simulink library "MotorLIB"  (R2019a)
settings: Solver=VariableStepAuto  StartTime=0.0  StopTime=10.0  RelTol=1e-3
libraries: fl_lib x5, nesl_utility x2, ee_lib x1
settings Model: Creator=plewi  LastModifiedBy=plewi

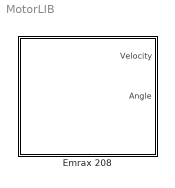
== system MotorLIB ==
  Emrax 208 : Subsystem  mask(Emrax 208){nPolePairs=10, pm_flux_linkage=0.05, Ld=125e-6, Lq=130e-6, L0=2e-4, Rs=0.35, J=256e3}
      mask prompts: nPolePairs "Number of pole pairs"; pm_flux_linkage "Permanent magnet flux linkage"; Ld "Stator d-axis inductance, Ld"; Lq "Stator q-axis inductance, Lq"; L0 "Stator zero-sequence inductance, L0"; Rs "Stator resistance per phase, Rs"; J "Rotor inertia (g cm^2)"
      mask help: Permanent Magnet Synchronous Motor with resolver attachment.
      mask TypeOptions nPolePairs:
      | Permanent Magnet
      | Synchronous Motor/nPolePairs
      mask TypeOptions pm_flux_linkage:
      | Permanent Magnet
      | Synchronous Motor/pm_flux_linkage
      mask TypeOptions Ld:
      | Permanent Magnet
      | Synchronous Motor/Ld
      mask TypeOptions Lq:
      | Permanent Magnet
      | Synchronous Motor/Lq
      mask TypeOptions L0:
      | Permanent Magnet
      | Synchronous Motor/L0
      mask TypeOptions Rs:
      | Permanent Magnet
      | Synchronous Motor/Rs
      mask TypeOptions J:
      | Permanent Magnet
      | Synchronous Motor/J
      mask Display: image('C:\Users\plewi\Documents\University\6-Sixth Year\MUR\MUR-E_Simulation_2019\Images\emrax_208_ip65_01-1-1024x1024.jpg');

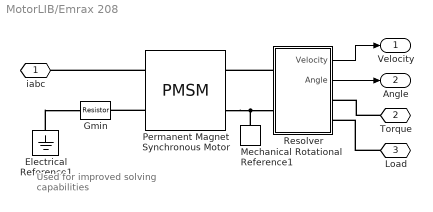
== system MotorLIB/Emrax 208 ==
  note: Used for improved
      | solving capabilities
  Electrical Reference1 : fl_lib/Electrical/Electrical Elements/Electrical Reference
  Gmin : fl_lib/Electrical/Electrical Elements/Resistor  R=1e9 Ohm  i_specify=off  i_priority=High  i=0 A  i_nominal_specify=off  i_nominal_unit=A  i_nominal_value=1  v_specify=off  v_priority=High  v=0 V  v_nominal_specify=off  v_nominal_unit=V  v_nominal_value=1
  Mechanical Rotational Reference1 : fl_lib/Mechanical/Rotational Elements/Mechanical Rotational Reference
  Permanent Magnet Synchronous Motor : ee_lib/Electromechanical/Permanent Magnet/PMSM  nPolePairs=nPolePairs  pmflux_param=1  pm_flux_linkage=pm_flux_linkage Wb  torque_constant=0.18 N*m/A  back_emf_constant=0.18 V/(rad/s)  stator_param=1  Ld=Ld H  Lq=Lq H  L0=L0 H  Ls=0.0002 H  Lm=0.00002 H  Ms=0.00002 H  Rs=Rs Ohm  zero_sequence=ee.enum.park.zerosequence.include  J=J g*cm^2  lam=0.01 N*m/(rad/s)  axes_param=ee.enum.rotorangle.qaxis  i_d_specify=off  i_d_priority=None  i_d=0 A  i_d_nominal_specify=off  i_d_nominal_unit=A  i_d_nominal_value=1  i_q_specify=off  i_q_priority=None  i_q=0 A  i_q_nominal_specify=off  i_q_nominal_unit=A  i_q_nominal_value=1  torque_specify=off  torque_priority=None  torque=0 N*m  torque_nominal_specify=off  torque_nominal_unit=N*m  torque_nominal_value=1  angular_velocity_specify=on  angular_velocity_priority=High  angular_velocity=0 rpm  angular_velocity_nominal_specify=off  angular_velocity_nominal_unit=rpm  angular_velocity_nominal_value=1  angular_position_specify=on  angular_position_priority=High  angular_position=0 rad  angular_position_nominal_specify=off  angular_position_nominal_unit=deg  angular_position_nominal_value=1  mask(PMSM){}
      settings: SourceProductName=Simscape Electrical
  Resolver : Subsystem
  iabc : PMIOPort  Side=Left
  Torque : PMIOPort  Port=2  Side=Right
  Load : PMIOPort  Port=3  Side=Left
  Velocity : Outport
  Angle : Outport  Port=2
  wires:
  Resolver/1(Velocity) -> Velocity/1
  Resolver/2(Angle) -> Angle/1
  connections:
  Electrical Reference1/LConn1 -- Gmin/LConn1
  Mechanical Rotational Reference1/LConn1 -- Permanent Magnet Synchronous Motor/RConn2 -- Resolver/LConn2
  Load/RConn1 -- Resolver/RConn2
  Permanent Magnet Synchronous Motor/LConn2 -- Gmin/RConn1
  Resolver/LConn1 -- Permanent Magnet Synchronous Motor/RConn1
  Permanent Magnet Synchronous Motor/LConn1 -- iabc/RConn1
  Torque/RConn1 -- Resolver/RConn1

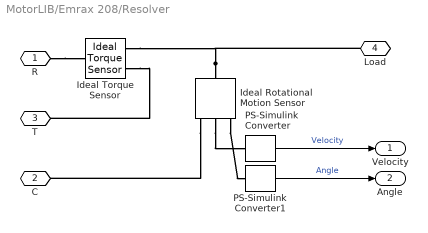
== system MotorLIB/Emrax 208/Resolver ==
  Ideal Rotational Motion Sensor : fl_lib/Mechanical/Mechanical Sensors/Ideal Rotational Motion Sensor  offset=0 deg
      settings: SourceProductName=Foundation Library
  Ideal Torque Sensor : fl_lib/Mechanical/Mechanical Sensors/Ideal Torque Sensor
      settings: SourceProductName=Foundation Library
  PS-Simulink Converter : nesl_utility/PS-Simulink Converter  PhysicalDomain=network_engine_domain  SubClassName=ps_output  LeftPortType=input  RightPortType=output  PseudoPeriodic=off  Frequencies=[]  Unit=rad/s  AffineConversion=off
  PS-Simulink Converter1 : nesl_utility/PS-Simulink Converter  PhysicalDomain=network_engine_domain  SubClassName=ps_output  LeftPortType=input  RightPortType=output  PseudoPeriodic=off  Frequencies=[]  Unit=rad  AffineConversion=off
  R : PMIOPort  Side=Left
  C : PMIOPort  Port=2  Side=Left
  T : PMIOPort  Port=3  Side=Right
  Load : PMIOPort  Port=4  Side=Right
  Velocity : Outport
  Angle : Outport  Port=2
  wires:
  PS-Simulink Converter1/1 -> Angle/1  "Angle"
  PS-Simulink Converter/1 -> Velocity/1  "Velocity"
  connections:
  Ideal Torque Sensor/RConn2 -- T/RConn1
  R/RConn1 -- Ideal Torque Sensor/LConn1
  Ideal Rotational Motion Sensor/RConn1 -- C/RConn1
  Ideal Rotational Motion Sensor/LConn1 -- Load/RConn1 -- Ideal Torque Sensor/RConn1
  Ideal Rotational Motion Sensor/RConn2 -- PS-Simulink Converter/LConn1
  Ideal Rotational Motion Sensor/RConn3 -- PS-Simulink Converter1/LConn1
